simulink model "swu_DIPC_6o_sim"  (R2023a)
settings: Solver=VariableStepAuto  StartTime=0.0  StopTime=5  FixedStep=1e-4  RelTol=1e-3
InitFcn:
  | m0=0.8; m1=0.5; m2=0.3; L1=0.3; L2=0.2; l1=0.15; l2=0.1; I1=0.006; I2=0.006; g=9.8;
  | d1=(m0+m1+m2);
  | d2=(m1*l1+m2*L1);
  | d3=m1*l1^2+m2*L1^2+I1;
  | d4=m2*l2;
  | d5=m2*L1*l2;
  | d6=m2*l2^2+I2;
settings Model: Creator=luand  LastModifiedBy=luand
settings SolverCC: ZeroCrossAlgorithm=Adaptive
settings DataIOCC: ReturnWorkspaceOutputs=off
settings DebuggingCC: MaxConsecutiveZCsMsg=warning
settings HardwareCC: ProdBitPerPointer=32  ProdBitPerSizeT=32  ProdBitPerPtrDiffT=32  ProdWordSize=32  ProdHWDeviceType=Intel->x86-32 (Windows32)

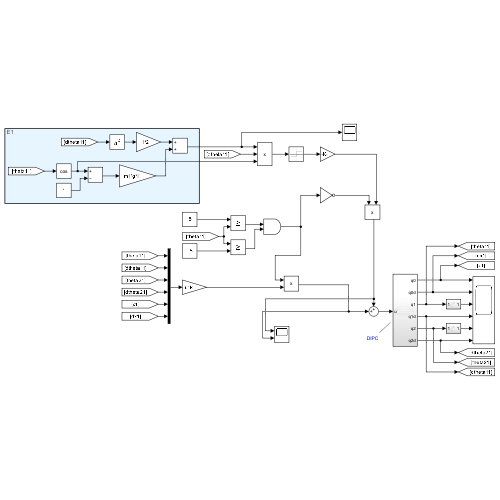
[thumbnail: Simulink's stored preview of the top-level diagram]
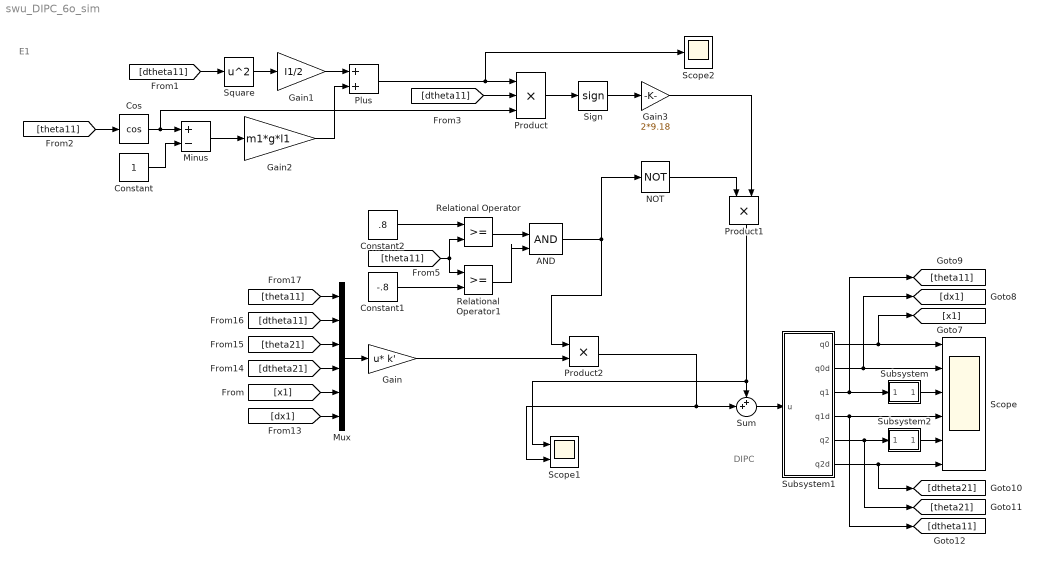
== system swu_DIPC_6o_sim ==
  note: E1
  note: DIPC
  AND : Logic  IconShape=distinctive  AllPortsSameDT=off  OutDataTypeStr=boolean
  Constant : Constant
  Constant1 : Constant  Value=-.8
  Constant2 : Constant  Value=.8
  Cos : Trigonometry  Operator=cos
  Gain : Gain  Gain=k'  Multiplication=Matrix(u*K)
  Gain1 : Gain  Gain=I1/2
  Gain2 : Gain  Gain=m1*g*l1
  Gain3 : Gain  Gain=2*9.18
  Minus : Sum  Inputs=+-
  Mux : Mux  Inputs=6
  NOT : Logic  Operator=NOT  IconShape=distinctive  AllPortsSameDT=off  OutDataTypeStr=boolean
  Plus : Sum
  Product : Product  Inputs=3
  Product1 : Product
  Product2 : Product
  Relational Operator : RelationalOperator  OutDataTypeStr=boolean  RndMeth=Simplest  InputSameDT=off
  Relational Operator1 : RelationalOperator  OutDataTypeStr=boolean  RndMeth=Simplest  InputSameDT=off
  Scope : Scope  NumInputPorts=6
  Scope1 : Scope  NumInputPorts=2
  Scope2 : Scope
  Sign : Signum
  Square : Math  Operator=square
  Subsystem : Subsystem
  Subsystem1 : Subsystem
  Subsystem2 : Subsystem
  Sum : Sum  Inputs=++|
  wires:
  Subsystem1/1(q0) -> Scope/1, [x1]
  Subsystem1/3(q1) -> Subsystem/1(In1), [theta11]
  Subsystem1/5(q2) -> Subsystem2/1(In1), [theta21]
  Subsystem1/2(q0d) -> Scope/2, [dx1]
  Subsystem1/6(q2d) -> [dtheta21], Scope/6
  Subsystem1/4(q1d) -> Scope/4, [dtheta11]
  [dx1] -> Mux/6
  [x1] -> Mux/5
  [dtheta11] -> Mux/2
  [theta11] -> Mux/1
  [dtheta21] -> Mux/4
  [theta21] -> Mux/3
  Gain1/1 -> Plus/1
  [dtheta11] -> Square/1
  Square/1 -> Gain1/1
  [theta11] -> Cos/1
  Cos/1 -> Product/3, Minus/1
  Constant/1 -> Minus/2
  Minus/1 -> Gain2/1
  Gain2/1 -> Plus/2
  Plus/1 -> Scope2/1, Product/1
  [dtheta11] -> Product/2
  Product/1 -> Sign/1
  Sign/1 -> Gain3/1
  Gain3/1 -> Product1/2
  Gain/1 -> Product2/2
  Sum/1 -> Subsystem1/1(u)
  Product1/1 -> Sum/1, Scope1/1
  Product2/1 -> Scope1/2, Sum/2
  Subsystem/1(Out1) -> Scope/3
  Subsystem2/1(Out1) -> Scope/5
  NOT/1 -> Product1/1
  Constant1/1 -> Relational Operator1/2
  [theta11] -> Relational Operator/2, Relational Operator1/1
  Relational Operator1/1 -> AND/2
  Relational Operator/1 -> AND/1
  AND/1 -> NOT/1, Product2/1
  Constant2/1 -> Relational Operator/1
  Mux/1 -> Gain/1

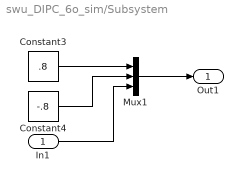
== system swu_DIPC_6o_sim/Subsystem ==
  In1 : Inport
  Constant3 : Constant  Value=.8
  Constant4 : Constant  Value=-.8
  Mux1 : Mux  Inputs=3
  Out1 : Outport
  wires:
  In1/1 -> Mux1/3
  Constant4/1 -> Mux1/2
  Constant3/1 -> Mux1/1
  Mux1/1 -> Out1/1

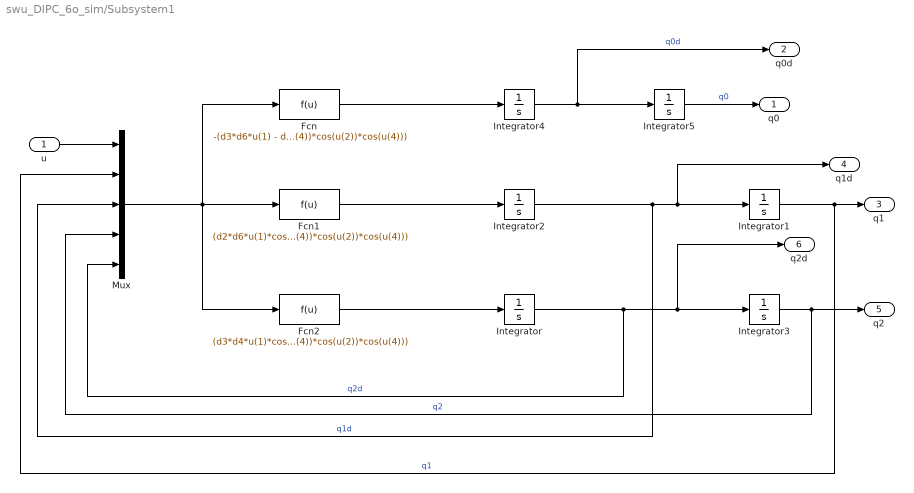
== system swu_DIPC_6o_sim/Subsystem1 ==
  u : Inport
  Fcn : Fcn  Expr=-(d3*d6*u(1) - d5^2*u(1)*cos(u(2) - u(4))^2 + d2*d3*d6*u(3)^2*sin(u(2)) + d3*d4*d6*u(5)^2*sin(u(4)) - d2*d5^2*u(3)^2*cos(u(2) - u(4))^2*sin(u(2)) - d4*d5^2*u(5)^2*cos(u(2) - u(4))^2*sin(u(4)) - d2^2*d6*g*cos(u(2))*sin(u(2)) - d3*d4^2*g*cos(u(4))*sin(u(4)) + d2*d5^2*u(3)^2*cos(u(2) - u(4))*sin(u(2) - u(4))*cos(u(2)) - d4*d5^2*u(5)^2*cos(u(2) - u(4))*sin(u(2) - u(4))*cos(u(4)) - d3*d4*d5*u(3)^2*sin(u(2) - u(4))*cos(u(4)) + d2*d5*d6*u(5)^2*sin(u(2) - u(4))*cos(u(2)) + d2*d4*d5*g*cos(u(2) - u(4))*cos(u(2))*sin(u(4)) + d2*d4*d5*g*cos(u(2) - u(4))*cos(u(4))*sin(u(2)))/(d3*d4^2*cos(u(4))^2 - d1*d3*d6 + d2^2*d6*cos(u(2))^2 + d1*d5^2*cos(u(2) - u(4))^2 - 2*d2*d4*d5*cos(u(2) - u(4))*cos(u(2))*cos(u(4)))
  Fcn1 : Fcn  Expr=(d2*d6*u(1)*cos(u(2)) + d2*d4^2*g*cos(u(4))^2*sin(u(2)) + d2^2*d6*u(3)^2*cos(u(2))*sin(u(2)) + d1*d5^2*u(3)^2*cos(u(2) - u(4))*sin(u(2) - u(4)) + d1*d5*d6*u(5)^2*sin(u(2) - u(4)) - d4*d5*u(1)*cos(u(2) - u(4))*cos(u(4)) - d4^2*d5*u(5)^2*sin(u(2) - u(4))*cos(u(4))^2 - d1*d2*d6*g*sin(u(2)) - d4^2*d5*u(5)^2*cos(u(2) - u(4))*cos(u(4))*sin(u(4)) + d2*d4*d6*u(5)^2*cos(u(2))*sin(u(4)) - d2*d4^2*g*cos(u(2))*cos(u(4))*sin(u(4)) + d1*d4*d5*g*cos(u(2) - u(4))*sin(u(4)) - d2*d4*d5*u(3)^2*cos(u(2) - u(4))*cos(u(4))*sin(u(2)) - d2*d4*d5*u(3)^2*sin(u(2) - u(4))*cos(u(2))*cos(u(4)))/(d3*d4^2*cos(u(4))^2 - d1*d3*d6 + d2^2*d6*cos(u(2))^2 + d1*d5^2*cos(u(2) - u(4))^2 - 2*d2*d4*d5*cos(u(2) - u(4))*cos(u(2))*cos(u(4)))
  Fcn2 : Fcn  Expr=(d3*d4*u(1)*cos(u(4)) + d2^2*d4*g*cos(u(2))^2*sin(u(4)) + d3*d4^2*u(5)^2*cos(u(4))*sin(u(4)) - d1*d5^2*u(5)^2*cos(u(2) - u(4))*sin(u(2) - u(4)) - d1*d3*d5*u(3)^2*sin(u(2) - u(4)) - d2*d5*u(1)*cos(u(2) - u(4))*cos(u(2)) + d2^2*d5*u(3)^2*sin(u(2) - u(4))*cos(u(2))^2 - d1*d3*d4*g*sin(u(4)) - d2^2*d5*u(3)^2*cos(u(2) - u(4))*cos(u(2))*sin(u(2)) + d2*d3*d4*u(3)^2*cos(u(4))*sin(u(2)) - d2^2*d4*g*cos(u(2))*cos(u(4))*sin(u(2)) + d1*d2*d5*g*cos(u(2) - u(4))*sin(u(2)) - d2*d4*d5*u(5)^2*cos(u(2) - u(4))*cos(u(2))*sin(u(4)) + d2*d4*d5*u(5)^2*sin(u(2) - u(4))*cos(u(2))*cos(u(4)))/(d3*d4^2*cos(u(4))^2 - d1*d3*d6 + d2^2*d6*cos(u(2))^2 + d1*d5^2*cos(u(2) - u(4))^2 - 2*d2*d4*d5*cos(u(2) - u(4))*cos(u(2))*cos(u(4)))
  Integrator{,2,4..5} (4 alike) : Integrator
  Integrator1 : Integrator  InitialCondition=-pi
  Integrator3 : Integrator  InitialCondition=-pi
  Mux : Mux  Inputs=5
  q0 : Outport  VectorParamsAs1DForOutWhenUnconnected=off
  q0d : Outport  Port=2  VectorParamsAs1DForOutWhenUnconnected=off
  q1 : Outport  Port=3  VectorParamsAs1DForOutWhenUnconnected=off
  q1d : Outport  Port=4  VectorParamsAs1DForOutWhenUnconnected=off
  q2 : Outport  Port=5  VectorParamsAs1DForOutWhenUnconnected=off
  q2d : Outport  Port=6  VectorParamsAs1DForOutWhenUnconnected=off
  wires:
  Integrator/1 -> Mux/5, q2d/1, Integrator3/1  "q2d"
  u/1 -> Mux/1
  Integrator1/1 -> Mux/2, q1/1  "q1"
  Integrator4/1 -> q0d/1, Integrator5/1  "q0d"
  Integrator5/1 -> q0/1  "q0"
  Integrator2/1 -> Mux/3, q1d/1, Integrator1/1  "q1d"
  Integrator3/1 -> Mux/4, q2/1  "q2"
  Mux/1 -> Fcn2/1, Fcn/1, Fcn1/1
  Fcn/1 -> Integrator4/1
  Fcn1/1 -> Integrator2/1
  Fcn2/1 -> Integrator/1

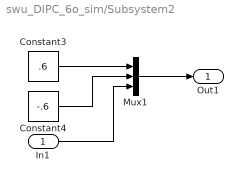
== system swu_DIPC_6o_sim/Subsystem2 ==
  In1 : Inport
  Constant3 : Constant  Value=.6
  Constant4 : Constant  Value=-.6
  Mux1 : Mux  Inputs=3
  Out1 : Outport
  wires:
  Mux1/1 -> Out1/1
  Constant3/1 -> Mux1/1
  Constant4/1 -> Mux1/2
  In1/1 -> Mux1/3
